simulink model "move_from_strain"  (R2017a)
settings: Solver=FixedStepDiscrete  StartTime=0.0  StopTime=inf  FixedStep=0.0002  RelTol=1e-3  EnableMultiTasking=on
libraries: xpcquanserlib x2, slrtlib x2, simulink x1
settings Model: SimulationMode=external  Creator=Venkatraman  LastModifiedBy=tbirdso
settings SolverCC: EnableConcurrentExecution=on
settings DataIOCC: LimitDataPoints=on  SaveFormat=Array  LoggingToFile=on
settings OptimizationCC: BlockReduction=off  OptimizeBlockIOStorage=off  BufferReuse=off  GlobalBufferReuse=off  ExpressionFolding=off  LocalBlockOutputs=off  LifeSpan=inf
settings DebuggingCC: SolverPrmCheckMsg=warning  SFUnexpectedBacktrackingDiag=warning  SFNoUnconditionalDefaultTransitionDiag=warning  SFExecutionAtInitializationDiag=none
settings HardwareCC: ProdBitPerPointer=32  ProdBitPerSizeT=32  ProdBitPerPtrDiffT=32  ProdLargestAtomicFloat=None  ProdWordSize=32  ProdLongLongMode=on  ProdHWDeviceType=Generic->32-bit x86 compatible  TargetBitPerPointer=64  TargetBitPerSizeT=64  TargetBitPerPtrDiffT=64  TargetLongLongMode=on  TargetIntDivRoundTo=Zero  TargetEndianess=LittleEndian  TargetWordSize=64  TargetHWDeviceType=MATLAB Host
settings ModelReferenceCC: PropagateSignalLabelsOutOfModel=off
settings RTWCC: SystemTargetFile=slrt.tlc  TemplateMakefile=slrt_default_tmf  Description=Simulink Real-Time  RTWVerbose=off  RTWCompilerOptimization=on
settings SimulinkRealTimeCC: GeneratePreprocessorConditionals=Disable all
settings ConfigComp: CovMetricSettings=dw  CovHtmlReporting=on  CovSaveCumulativeToWorkspaceVar=on  CovSaveSingleToWorkspaceVar=on  CovExternalEMLEnable=off  CovSFcnEnable=off

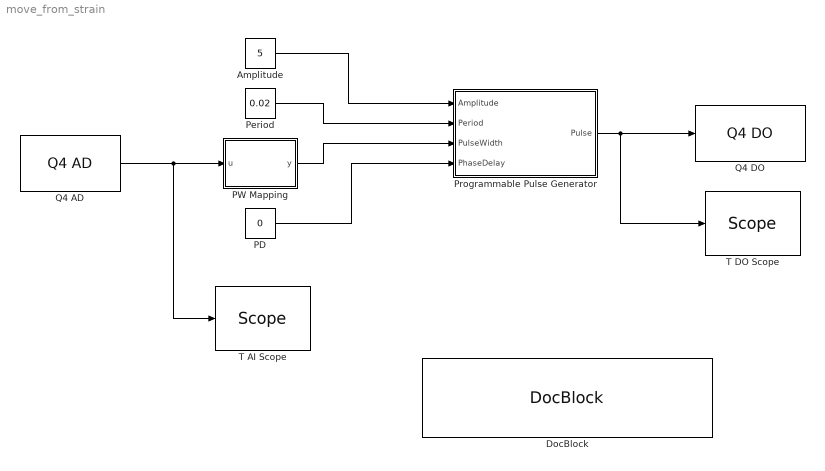
== system move_from_strain ==
  Amplitude : Constant  Value=5
  DocBlock : simulink/Model-Wide Utilities/DocBlock  DocumentType=Text
      content=|
      | TO LOG SIGNAL DATA:
      | 1) Run the project
      | 2) Open "Simulation Data Inspector"
      | 3) Choose the signals you want to log
      | 4) Stop the simulation
      | 5) Select "export" and give signals a name
      | 6) In MATLAB workspace run "plot([yourname])"
      |
      | TO LOG A NEW SIGNAL
      | 1) Right click signal
      | 2) Select "Log Selected Signal"
  PD : Constant  Value=0
  PW Mapping : MATLAB Function  TreatAsAtomicUnit=on
  Period : Constant  Value=0.02
  Programmable Pulse Generator : Subsystem
  Q4 AD : xpcquanserlib/A//D/Q4 AD  channel=[1]  sampleTime=0.0002  slot=-1
      settings: SourceProductName=Simulink Real-Time  SourceProductBaseCode=XP
  "Q4 DO " : xpcquanserlib/Digital Output/Q4 DO   channel=[1]  reset=[1]  initValue=[0]  sampleTime=.0002  slot=-1
      settings: SourceProductName=Simulink Real-Time  SourceProductBaseCode=XP
  T AI Scope : slrtlib/Displays and Logging/Scope   scopeno=2  scopetype=Target  autostart=on  viewmode=Graphical redraw  formatstr='%15.6f'  grid=on  ylimits=[0, 2]  nosamples=250  noprepostsamples=0  interleave=1  triggermode=FreeRun  triggersignal=1  trigsignalfromport=off  triggerlevel=0.0  triggerslope=Either  triggerscope=1  triggersample=0  filename=data.dat  mode=Lazy  writesize=512  autorestart=off  dynamicfilemode=off  maxwritefilesize=512*1024^2
  T DO Scope : slrtlib/Displays and Logging/Scope   scopeno=1  scopetype=Target  autostart=on  viewmode=Graphical redraw  formatstr='%15.6f'  grid=on  ylimits=[0, 6]  nosamples=250  noprepostsamples=0  interleave=1  triggermode=FreeRun  triggersignal=1  trigsignalfromport=off  triggerlevel=0.0  triggerslope=Either  triggerscope=1  triggersample=0  filename=data.dat  mode=Lazy  writesize=512  autorestart=off  dynamicfilemode=off  maxwritefilesize=512*1024^2
  wires:
  PW Mapping/1(y) -> Programmable Pulse Generator/3(PulseWidth)
  Period/1 -> Programmable Pulse Generator/2(Period)
  Amplitude/1 -> Programmable Pulse Generator/1(Amplitude)
  PD/1 -> Programmable Pulse Generator/4(PhaseDelay)
  Programmable Pulse Generator/1(Pulse) -> "Q4 DO "/1, T DO Scope/1
  Q4 AD/1 -> T AI Scope/1, PW Mapping/1(u)

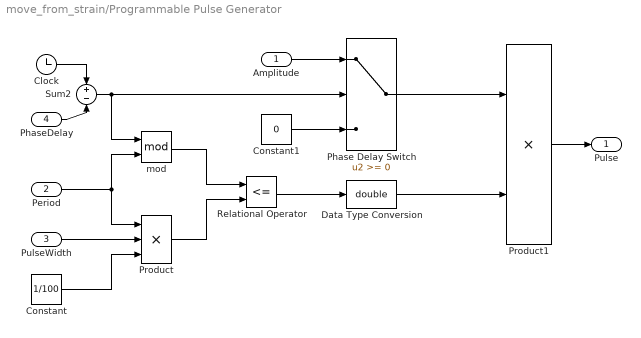
== system move_from_strain/Programmable Pulse Generator ==
  Amplitude : Inport
  Period : Inport  Port=2
  PulseWidth : Inport  Port=3
  PhaseDelay : Inport  Port=4
  Clock : Clock
  Constant : Constant  Value=1/100
  Constant1 : Constant  Value=0
  Data Type Conversion : DataTypeConversion  OutDataTypeStr=double
  Phase Delay Switch : Switch
  Product : Product  Inputs=3  RndMeth=Zero
  Product1 : Product  RndMeth=Zero
  Relational Operator : RelationalOperator  Operator=<=  RndMeth=Nearest
  Sum2 : Sum  Inputs=+-
  mod : Math  Operator=mod  SaturateOnIntegerOverflow=on
  Pulse : Outport
  wires:
  Phase Delay Switch/1 -> Product1/1
  Constant1/1 -> Phase Delay Switch/3
  Amplitude/1 -> Phase Delay Switch/1
  Sum2/1 -> Phase Delay Switch/2, mod/1
  PhaseDelay/1 -> Sum2/2
  Clock/1 -> Sum2/1
  Period/1 -> mod/2, Product/1
  mod/1 -> Relational Operator/1
  PulseWidth/1 -> Product/2
  Constant/1 -> Product/3
  Relational Operator/1 -> Data Type Conversion/1
  Data Type Conversion/1 -> Product1/2
  Product1/1 -> Pulse/1
  Product/1 -> Relational Operator/2

== matlab function move_from_strain/PW Mapping ==
  data: u input; y output
function y = fcn(u)

y = floor(u)*10 + 2.2;
